simulink model "Task_1"  (R2023a)
settings: Solver=VariableStepAuto  StartTime=0.0  StopTime=0  RelTol=1e-3
undefined symbols (not defined in the file or in its folder): Rec, SDTV
libraries: visionsinks x2, dspstat3 x2, visionconversions x1, visionanalysis x1, visionsources x1
settings Model: Creator=alexa  LastModifiedBy=davidmarafuzgaspar
settings DebuggingCC: UnconnectedInputMsg=warning  UnconnectedOutputMsg=warning  UnconnectedLineMsg=warning
settings ModelReferenceCC: EnableRefExpFcnMdlSchedulingChecks=on
settings RTWCC: DLArmComputeVersion=19.05

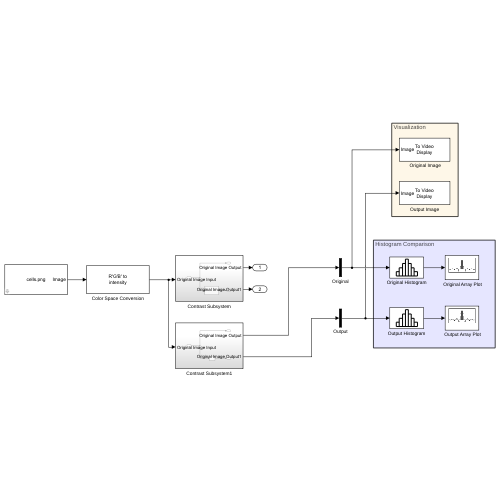
[thumbnail: Simulink's stored preview of the top-level diagram]
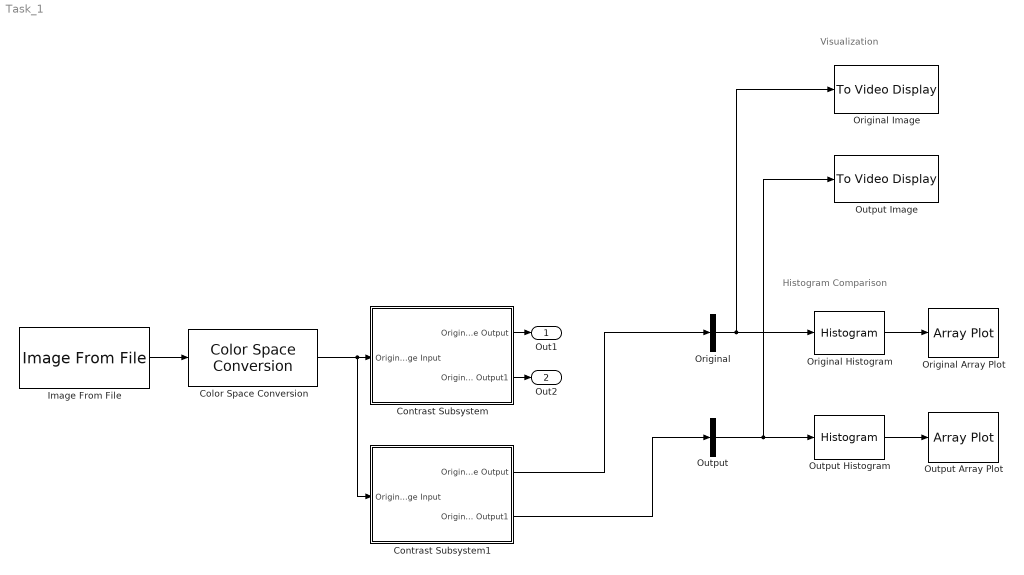
== system Task_1 ==
  note: Visualization
  note: Histogram Comparison
  " Original Array Plot" : ArrayPlot  ScopeFrameLocation=window
  " Original Image" : visionsinks/To Video Display  windowSizeMode=Normal  openAtMdlStart=on  fullScreen=off  videoWindowX=815  videoWindowY=-1455  saveWindowSize=off  videoWindowWidth=854  videoWindowHeight=872  inputColorFormat=RGB  inputType=Obsolete  imagePorts=One multidimensional signal  OutputDevice=On-screen video monitor  dataOrg=Column-major  isWindowOpen=on
  " Output Array Plot" : ArrayPlot  ScopeFrameLocation=window
  Color Space Conversion : visionconversions/Color Space  Conversion  conversion=Obsolete  conversionActive=R'G'B' to intensity  wp_str=D65  rec=Rec. 601 (SDTV)  sys=1125/60/2:1  imagePorts=One multidimensional signal
  Contrast Subsystem : Subsystem
  Contrast Subsystem1 : Subsystem
  Image From File : visionsources/Image From File  Tag=vipblks_nd  FileName=/home/davidmarafuzgaspar/Desktop/ist-computational-vision-project/Lab 3/Data/cells.png  Ts=0.1  imagePorts=One multidimensional signal  OutPortLabels=R|G|B  ImageDataType=double  sdImageDataType=uint(8)  Signed=on  WordLength=16  FractionLengthMode=User-defined  FractionLength=15
  Original : Mux  Inputs=1
  Original Histogram : dspstat3/Histogram  umin=0  umax=255  nbins=255  operateOver=Each column  Dimension=1  normalized=off  run=off  reset=on  trigtype=Non-zero sample  colComp=on  roundingMode=Floor  overflowMode=off
  Output : Mux  Inputs=1
  Output Histogram : dspstat3/Histogram  umin=0  umax=255  nbins=255  operateOver=Each column  Dimension=1  normalized=off  run=off  reset=on  trigtype=Non-zero sample  colComp=on  roundingMode=Floor  overflowMode=off
  Output Image : visionsinks/To Video Display  windowSizeMode=Normal  openAtMdlStart=on  fullScreen=off  videoWindowX=1713  videoWindowY=-1322  saveWindowSize=off  videoWindowWidth=854  videoWindowHeight=872  inputColorFormat=RGB  inputType=Obsolete  imagePorts=One multidimensional signal  OutputDevice=On-screen video monitor  dataOrg=Column-major  isWindowOpen=on
  Out1 : Outport
  Out2 : Outport  Port=2
  wires:
  Image From File/1 -> Color Space Conversion/1
  Color Space Conversion/1 -> Contrast Subsystem1/1(Original Image Input), Contrast Subsystem/1(Original Image Input)
  Original Histogram/1 -> " Original Array Plot"/1
  Output Histogram/1 -> " Output Array Plot"/1
  Original/1 -> Original Histogram/1, " Original Image"/1
  Output/1 -> Output Histogram/1, Output Image/1
  Contrast Subsystem1/1(Original Image Output) -> Original/1
  Contrast Subsystem1/2(Original Image Output1) -> Output/1
  Contrast Subsystem/1(Original Image Output) -> Out1/1
  Contrast Subsystem/2(Original Image Output1) -> Out2/1

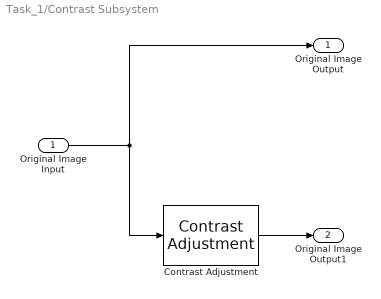
== system Task_1/Contrast Subsystem ==
  Original Image Input : Inport
  Contrast Adjustment : visionanalysis/Contrast Adjustment  methodInputRange=Full input data range [min max]  rangeIn=[0 255]  fracSaturate=[1 1]  isBinNum=on  binNum=256  methodOutputRange=Full data type range  rangeOut=[0 255]  roundingMode=Floor  overflowMode=off  prod1Mode=Binary point scaling  prod1WordLength=32  prod1FracLength=16  prod2Mode=Binary point scaling  prod2WordLength=32  prod2FracLength=16
  Original Image Output : Outport
  Original Image Output1 : Outport  Port=2
  wires:
  Original Image Input/1 -> Contrast Adjustment/1, Original Image Output/1
  Contrast Adjustment/1 -> Original Image Output1/1

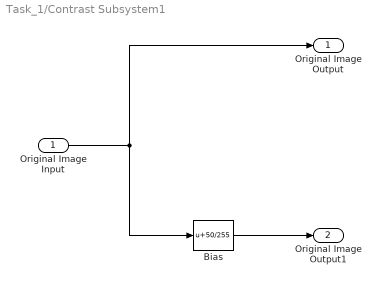
== system Task_1/Contrast Subsystem1 ==
  Original Image Input : Inport
  Bias : Bias  Bias=50/255  SaturateOnIntegerOverflow=off
  Original Image Output : Outport
  Original Image Output1 : Outport  Port=2
  wires:
  Original Image Input/1 -> Bias/1, Original Image Output/1
  Bias/1 -> Original Image Output1/1
